simulink library "pbd"  (Simulink 8.1)
settings: Solver=ode1  StartTime=0.0  StopTime=Inf  FixedStep=0.001  RelTol=1e-3
PostLoadFcn:
  | , if any(exist('dsrtsu_mdlpostloadfcn', 'file') == [2, 3, 6]), try dsrtsu_mdlpostloadfcn('Execute', bdroot); catch fprintf('Error in PostLoadFcn (dsrtsu_mdlpostloadfcn) for model "%s":\n %s\n', bdroot, lasterr); end, end,
undefined symbols (not defined in the file or in its folder): KACC_ACCBrakeDisableSpd_kph, KACC_ACCRelSpdDistThreshold_kph, KACC_ACCRelSpdThreshold_kph, KACC_ACCTGapMargin_s, KACC_BrakeDisableDist_m
libraries: hcu_lib x3
settings Model: DSRTSU_INTERNAL_RTI_VER=450  DSRTSU_INTERNAL_RTI_TYPE=rti1401  RTICANMMDATA=struct('GeneralSetupData',struct('modelroot','D:\ELN150201_TAIWAN\trunk\AdasDragon\software\sw_development\arch\app\acc','generalsettings',struct('filesettings',struct('destfolder',struct('Name','RTICANMM_FILES','Check',1),'buildfolder',struct('Name','.','Check',1),'AbsDestfolder',struct('Name','D:\ELN150201_TAIWAN\trunk\AdasDragon\software\sw_development\arch\app\acc\RTICANMM_FILES'),'AbsBuildfolder',struct('Name','D:\ELN150201_TAIWAN\trunk\AdasDragon\software\sw_development\arch\app\acc'))),'options',struct('addpaths',1,'rmpaths',1,'addtrcexclusion',logical(1),'cannavigator',struct('checkmonitoring',0),'show_usrtrc',0,'use_usrtrc',0),'advanced',struct('options',[1 1 1 1 1 1 1 1 1 1 1 1 1 1 1 1 1 1 1 1 1 1 1 1 1 1 1 1 1 1 1 1 1 1 1 1 1 1 1 1 1 1 1 1 1 1 1 1 1 1 1 1 1 1 1 1 1 1 1 1 1 1 1 1 1 1 1 1 1 1 1 1 1 1 1 1 1 1 1 1 1 1 1 1 1 1 1 1 1 1 1 1 1 1 1 1 1 1 1 1]),'MPSetup',{{}},'modelname','pbd','block','pbd'))  DSRTSU_INTERNAL_RTIFPGA=40  Creator=AT015555  LastModifiedBy=AT015555

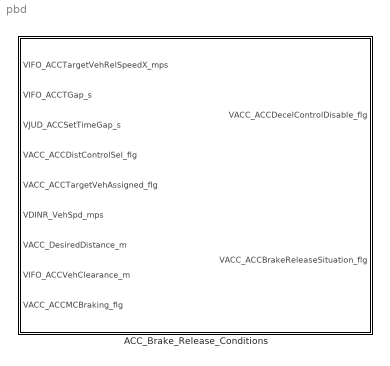
== system pbd ==
  ACC_Brake_Release_Conditions : Subsystem

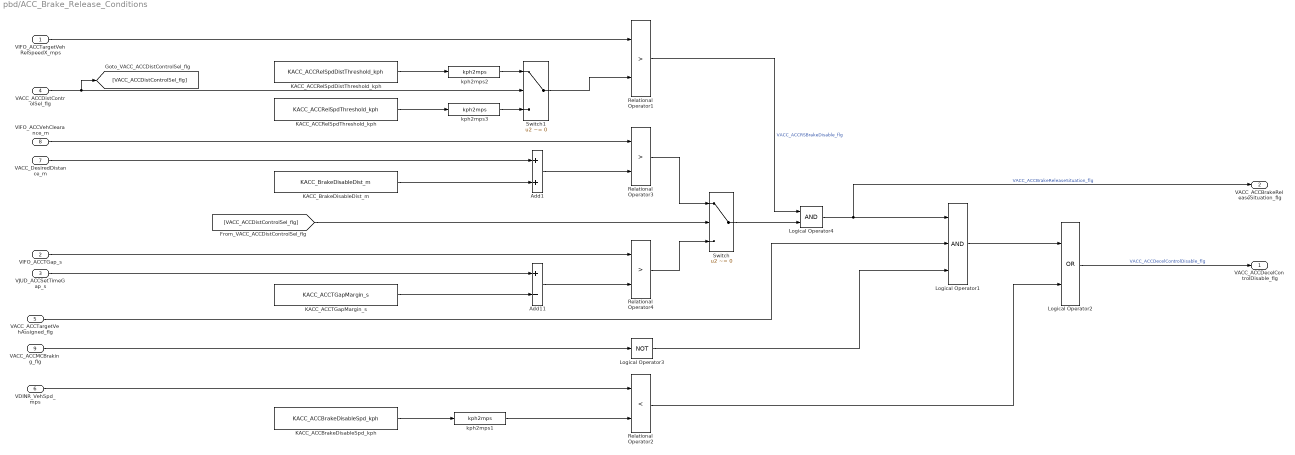
== system pbd/ACC_Brake_Release_Conditions ==
  VIFO_ACCTargetVehRelSpeedX_mps : Inport
  VIFO_ACCTGap_s : Inport  Port=2
  VJUD_ACCSetTimeGap_s : Inport  Port=3
  VACC_ACCDistControlSel_flg : Inport  Port=4
  VACC_ACCTargetVehAssigned_flg : Inport  Port=5
  VDINR_VehSpd_mps : Inport  Port=6
  VACC_DesiredDistance_m : Inport  Port=7
  VIFO_ACCVehClearance_m : Inport  Port=8
  VACC_ACCMCBraking_flg : Inport  Port=9
  Add1 : Sum
  Add11 : Sum  Inputs=+-
  KACC_ACCBrakeDisableSpd_kph : Constant  Value=KACC_ACCBrakeDisableSpd_kph
  KACC_ACCRelSpdDistThreshold_kph : Constant  Value=KACC_ACCRelSpdDistThreshold_kph
  KACC_ACCRelSpdThreshold_kph : Constant  Value=KACC_ACCRelSpdThreshold_kph
  KACC_ACCTGapMargin_s : Constant  Value=KACC_ACCTGapMargin_s
  KACC_BrakeDisableDist_m : Constant  Value=KACC_BrakeDisableDist_m
  Logical Operator1 : Logic  Inputs=3  AllPortsSameDT=off  OutDataTypeStr=boolean
  Logical Operator2 : Logic  Operator=OR  AllPortsSameDT=off  OutDataTypeStr=boolean
  Logical Operator3 : Logic  Operator=NOT  Inputs=3  AllPortsSameDT=off  OutDataTypeStr=boolean
  Logical Operator4 : Logic  AllPortsSameDT=off  OutDataTypeStr=boolean
  Relational Operator1 : RelationalOperator  Operator=>  OutDataTypeStr=boolean
  Relational Operator2 : RelationalOperator  Operator=<  OutDataTypeStr=boolean
  Relational Operator3 : RelationalOperator  Operator=>  OutDataTypeStr=boolean
  Relational Operator4 : RelationalOperator  Operator=>  OutDataTypeStr=boolean
  Switch : Switch  Criteria=u2 ~= 0
  Switch1 : Switch  Criteria=u2 ~= 0
  kph2mps1 : hcu_lib/kph2mps
  kph2mps2 : hcu_lib/kph2mps
  kph2mps3 : hcu_lib/kph2mps
  VACC_ACCDecelControlDisable_flg : Outport
  VACC_ACCBrakeReleaseSituation_flg : Outport  Port=2
  wires:
  Logical Operator2/1 -> VACC_ACCDecelControlDisable_flg/1  "VACC_ACCDecelControlDisable_flg"
  Relational Operator1/1 -> Logical Operator4/1  "VACC_ACCRSBrakeDisable_flg"
  kph2mps3/1 -> Switch1/3
  VIFO_ACCTargetVehRelSpeedX_mps/1 -> Relational Operator1/1
  KACC_ACCRelSpdThreshold_kph/1 -> kph2mps3/1
  KACC_ACCTGapMargin_s/1 -> Add11/2
  Add11/1 -> Relational Operator4/2
  VACC_ACCTargetVehAssigned_flg/1 -> Logical Operator1/2
  Logical Operator1/1 -> Logical Operator2/1
  VDINR_VehSpd_mps/1 -> Relational Operator2/1
  KACC_ACCBrakeDisableSpd_kph/1 -> kph2mps1/1
  kph2mps1/1 -> Relational Operator2/2
  Relational Operator2/1 -> Logical Operator2/2
  VIFO_ACCTGap_s/1 -> Relational Operator4/1
  VJUD_ACCSetTimeGap_s/1 -> Add11/1
  KACC_BrakeDisableDist_m/1 -> Add1/2
  Add1/1 -> Relational Operator3/2
  VACC_DesiredDistance_m/1 -> Add1/1
  Switch/1 -> Logical Operator4/2
  VIFO_ACCVehClearance_m/1 -> Relational Operator3/1
  Relational Operator3/1 -> Switch/1
  VACC_ACCDistControlSel_flg/1 -> [VACC_ACCDistControlSel_flg], Switch1/2
  Relational Operator4/1 -> Switch/3
  KACC_ACCRelSpdDistThreshold_kph/1 -> kph2mps2/1
  kph2mps2/1 -> Switch1/1
  Switch1/1 -> Relational Operator1/2
  [VACC_ACCDistControlSel_flg] -> Switch/2
  VACC_ACCMCBraking_flg/1 -> Logical Operator3/1
  Logical Operator3/1 -> Logical Operator1/3
  Logical Operator4/1 -> VACC_ACCBrakeReleaseSituation_flg/1, Logical Operator1/1  "VACC_ACCBrakeReleaseSituation_flg"
